simulink model "BAL_test"  (Simulink 7.4)
settings: Solver=FixedStepDiscrete  StartTime=0.0  StopTime=10  FixedStep=0.01  RelTol=1e-3
libraries: BAL_lib x1, simulink x1
settings Model: Creator=Administrator  LastModifiedBy=sunsijun
settings DataIOCC: SaveFormat=Structure
settings OptimizationCC: InitFltsAndDblsToZero=on
settings DebuggingCC: InheritedTsInSrcMsg=none  ParameterPrecisionLossMsg=none
settings RTWCC: GenCodeOnly=on

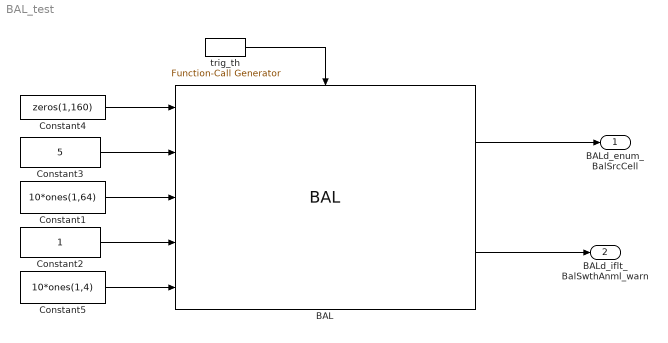
== system BAL_test ==
  BAL : BAL_lib/BAL  SystemSampleTime=-1
  Constant1 : Constant  Value=10*ones(1,64)  OutDataTypeMode=single  OutDataType=fixdt(1, 16)  OutScaling=2^0  OutDataTypeStr=single
  Constant2 : Constant  OutDataTypeMode=uint8  OutDataType=fixdt(1, 16)  OutScaling=2^0  OutDataTypeStr=uint8
  Constant3 : Constant  Value=5  OutDataTypeMode=uint8  OutDataType=fixdt(1, 16)  OutScaling=2^0  OutDataTypeStr=uint8
  Constant4 : Constant  Value=zeros(1,160)  OutDataTypeMode=single  OutDataType=fixdt(1, 16)  OutScaling=2^0  OutDataTypeStr=single
  Constant5 : Constant  Value=10*ones(1,4)  OutDataTypeMode=single  OutDataType=fixdt(1, 16)  OutScaling=2^0  OutDataTypeStr=single
  trig_th : simulink/Ports & Subsystems/Function-Call Generator  sample_time=-1  numberOfIterations=1
  BALd_enum_BalSrcCell : Outport
  BALd_iflt_BalSwthAnml_warn : Outport  Port=2  OutDataType=fixdt(1, 16)  OutScaling=2^0
  wires:
  trig_th/1 -> BAL/Trigger
  BAL/1 -> BALd_enum_BalSrcCell/1
  BAL/2 -> BALd_iflt_BalSwthAnml_warn/1
  Constant4/1 -> BAL/1
  Constant3/1 -> BAL/2
  Constant1/1 -> BAL/3
  Constant2/1 -> BAL/4
  Constant5/1 -> BAL/5
